simulink model "feedbackcontrol2"  (R2017b)
settings: Solver=VariableStepAuto  StartTime=0.0  StopTime=2000  MaxStep=0.04  RelTol=1e-3
values from neighbouring files (symbols this model uses):
  azi0 = 90/180*pi    (= 1.57079632679)    [MonteCarlo_f.m]    (also in MonteCarlo_l.m; MonteCarlo_s.m; calcu_delta.m = 0.174532925199; calcu_delta11.m)
  cd0 = 0.024    [flight_sim.m]
  cd1 = 7.24e-4    (= 0.000724)    [flight_sim.m]
  cd2 = 0.406    [flight_sim.m]
  cl0 = -0.2317    [flight_sim.m]
  cl1 = 0.0513    [flight_sim.m]
  cl2 = 0.2945    [flight_sim.m]
  delta_d = delta_d0(ii)    [MonteCarlo_f.m]    (also in MonteCarlo_l.m; MonteCarlo_s.m; calcu_delta11.m = -0.08; calcu_delta3.m = -0.079)
  delta_l = delta_l0(ii)    [MonteCarlo_f.m]    (also in MonteCarlo_l.m; MonteCarlo_s.m; calcu_delta3.m = 0.05)
  fpa0 = theta_0(ii)    [MonteCarlo_f.m]    (also in MonteCarlo_l.m; MonteCarlo_s.m; calcu_delta.m = -0.0349065850399; calcu_delta11.m = -0.0349065850399)
  hs = 7320    [constant.m]    (also in flight_sim.m)
  lat0 = 0    [MonteCarlo_f.m]    (also in MonteCarlo_l.m; MonteCarlo_s.m; calcu_delta.m; calcu_delta11.m)
  lon0 = 0    [MonteCarlo_f.m]    (also in MonteCarlo_l.m; MonteCarlo_s.m; calcu_delta.m; calcu_delta11.m)
  m = 92079.25    [constant.m]    (also in flight_sim.m = 907.2)
  r0 = r_0(ii)    [MonteCarlo_f.m]    (also in MonteCarlo_l.m; MonteCarlo_s.m; calcu_delta.m = Re+97500; calcu_delta11.m = Re+100000)
  Re = 6371393    [calcu_R.m]    (also in calcu_R2.m; calcu_c.m; constant.m = 6378145; flight_sim.m)
  rho0 = rho_0(ii)    [MonteCarlo_f.m]    (also in MonteCarlo_l.m; MonteCarlo_s.m; constant.m = 1.225; flight_sim.m = 1.225)
  S = 249.9    [constant.m]    (also in flight_sim.m = 0.484)
  solution = output.result.solution    [calcu_A_B.m]    (also in calcu_A_B1.m; calcu_A_B2.m; main_bank.m)
  V0 = V_0(ii)    [MonteCarlo_f.m]    (also in MonteCarlo_l.m; MonteCarlo_s.m; calcu_delta.m = 7900; calcu_delta11.m = 7900)
undefined symbols (not defined in the file or in its folder): Kdh, Kh, mu
settings Model: NumberOfSteps=500  Creator=ztyab  LastModifiedBy=ztyab
settings DataIOCC: SaveFormat=Array

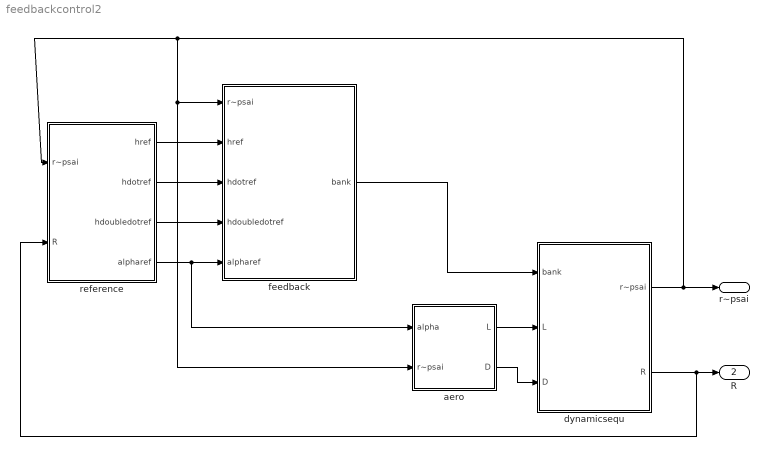
== system feedbackcontrol2 ==
  aero : Subsystem
  dynamicsequ : Subsystem
  feedback : Subsystem
  reference : Subsystem
  r~psai : Outport
  R : Outport  Port=2
  wires:
  aero/1(L) -> dynamicsequ/2(L)
  aero/2(D) -> dynamicsequ/3(D)
  reference/4(alpharef) -> aero/1(alpha), feedback/5(alpharef)
  reference/3(hdoubledotref) -> feedback/4(hdoubledotref)
  reference/1(href) -> feedback/2(href)
  reference/2(hdotref) -> feedback/3(hdotref)
  dynamicsequ/2(R) -> reference/2(R), R/1
  dynamicsequ/1(r~psai) -> feedback/1(r~psai), aero/2(r~psai), reference/1(r~psai), r~psai/1
  feedback/1(bank) -> dynamicsequ/1(bank)

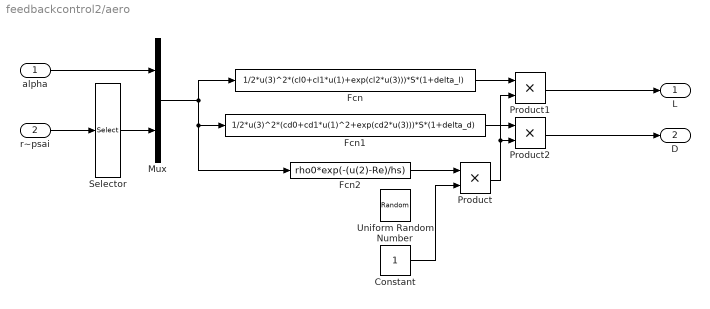
== system feedbackcontrol2/aero ==
  alpha : Inport
  r~psai : Inport  Port=2
  Constant : Constant
  Fcn : Fcn  Expr=1/2*u(3)^2*(cl0+cl1*u(1)+exp(cl2*u(3)))*S*(1+delta_l)
  Fcn1 : Fcn  Expr=1/2*u(3)^2*(cd0+cd1*u(1)^2+exp(cd2*u(3)))*S*(1+delta_d)
  Fcn2 : Fcn  Expr=rho0*exp(-(u(2)-Re)/hs)
  Mux : Mux  Inputs=2
  Product : Product
  Product1 : Product
  Product2 : Product
  Selector : Selector  InputPortWidth=6  IndexOptions=Index vector (dialog)  Indices=[1 4]  OutputSizes=1
  Uniform Random Number : UniformRandomNumber  Minimum=0.5  Maximum=1.5  SampleTime=0.01
  L : Outport
  D : Outport  Port=2
  wires:
  Mux/1 -> Fcn1/1, Fcn2/1, Fcn/1
  alpha/1 -> Mux/1
  r~psai/1 -> Selector/1
  Selector/1 -> Mux/2
  Fcn2/1 -> Product/1
  Product/1 -> Product1/2, Product2/2
  Fcn/1 -> Product1/1
  Fcn1/1 -> Product2/1
  Product1/1 -> L/1
  Product2/1 -> D/1
  Constant/1 -> Product/2

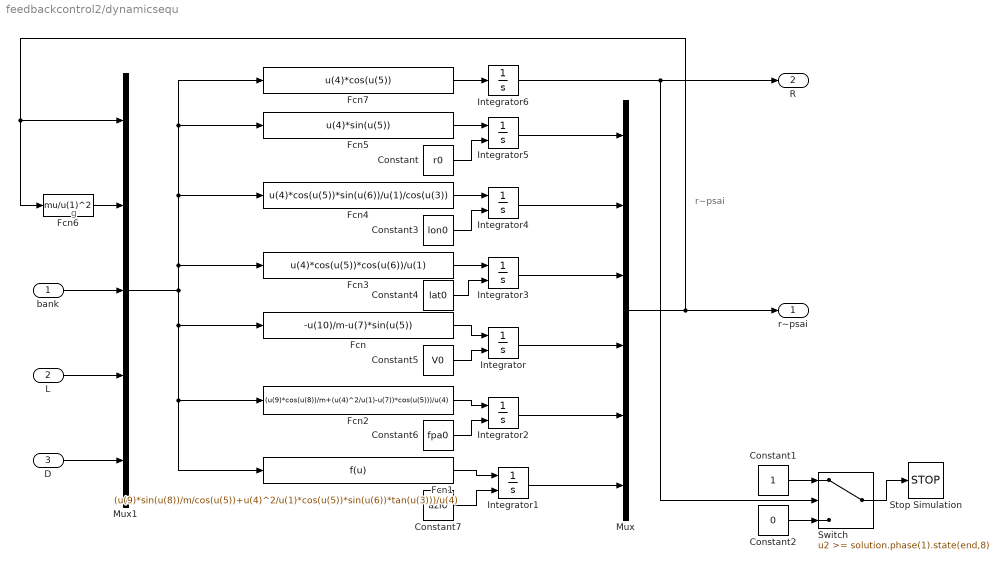
== system feedbackcontrol2/dynamicsequ ==
  note: g
  note: r~psai
  bank : Inport
  L : Inport  Port=2
  D : Inport  Port=3
  Constant : Constant  Value=r0
  Constant1 : Constant
  Constant2 : Constant  Value=0
  Constant3 : Constant  Value=lon0
  Constant4 : Constant  Value=lat0
  Constant5 : Constant  Value=V0
  Constant6 : Constant  Value=fpa0
  Constant7 : Constant  Value=azi0
  Fcn : Fcn  Expr=-u(10)/m-u(7)*sin(u(5))
  Fcn1 : Fcn  Expr=(u(9)*sin(u(8))/m/cos(u(5))+u(4)^2/u(1)*cos(u(5))*sin(u(6))*tan(u(3)))/u(4)
  Fcn2 : Fcn  Expr=(u(9)*cos(u(8))/m+(u(4)^2/u(1)-u(7))*cos(u(5)))/u(4)
  Fcn3 : Fcn  Expr=u(4)*cos(u(5))*cos(u(6))/u(1)
  Fcn4 : Fcn  Expr=u(4)*cos(u(5))*sin(u(6))/u(1)/cos(u(3))
  Fcn5 : Fcn  Expr=u(4)*sin(u(5))
  Fcn6 : Fcn  Expr=mu/u(1)^2
  Fcn7 : Fcn  Expr=u(4)*cos(u(5))
  Integrator : Integrator  InitialConditionSource=external  InitialCondition=7500
  Integrator1 : Integrator  InitialConditionSource=external  InitialCondition=10*pi/180
  Integrator2 : Integrator  InitialConditionSource=external  InitialCondition=-2/180*pi
  Integrator3 : Integrator  InitialConditionSource=external
  Integrator4 : Integrator  InitialConditionSource=external
  Integrator5 : Integrator  InitialConditionSource=external  InitialCondition=95000+6371393
  Integrator6 : Integrator
  Mux : Mux  Inputs=6
  Mux1 : Mux  Inputs=5
  Stop Simulation : Stop
  Switch : Switch  Threshold=solution.phase(1).state(end,8)
  r~psai : Outport
  R : Outport  Port=2
  wires:
  Fcn6/1 -> Mux1/2
  Mux/1 -> Fcn6/1, Mux1/1, r~psai/1
  Fcn1/1 -> Integrator1/1
  Integrator1/1 -> Mux/6
  Fcn2/1 -> Integrator2/1
  Integrator4/1 -> Mux/2
  Fcn/1 -> Integrator/1
  Integrator2/1 -> Mux/5
  Fcn4/1 -> Integrator4/1
  Integrator3/1 -> Mux/3
  Fcn3/1 -> Integrator3/1
  Integrator/1 -> Mux/4
  Fcn5/1 -> Integrator5/1
  Integrator5/1 -> Mux/1
  L/1 -> Mux1/4
  D/1 -> Mux1/5
  bank/1 -> Mux1/3
  Mux1/1 -> Fcn1/1, Fcn2/1, Fcn/1, Fcn4/1, Fcn7/1, Fcn5/1, Fcn3/1
  Fcn7/1 -> Integrator6/1
  Integrator6/1 -> Switch/2, R/1
  Constant2/1 -> Switch/3
  Constant1/1 -> Switch/1
  Switch/1 -> Stop Simulation/1
  Constant/1 -> Integrator5/2
  Constant3/1 -> Integrator4/2
  Constant4/1 -> Integrator3/2
  Constant5/1 -> Integrator/2
  Constant6/1 -> Integrator2/2
  Constant7/1 -> Integrator1/2

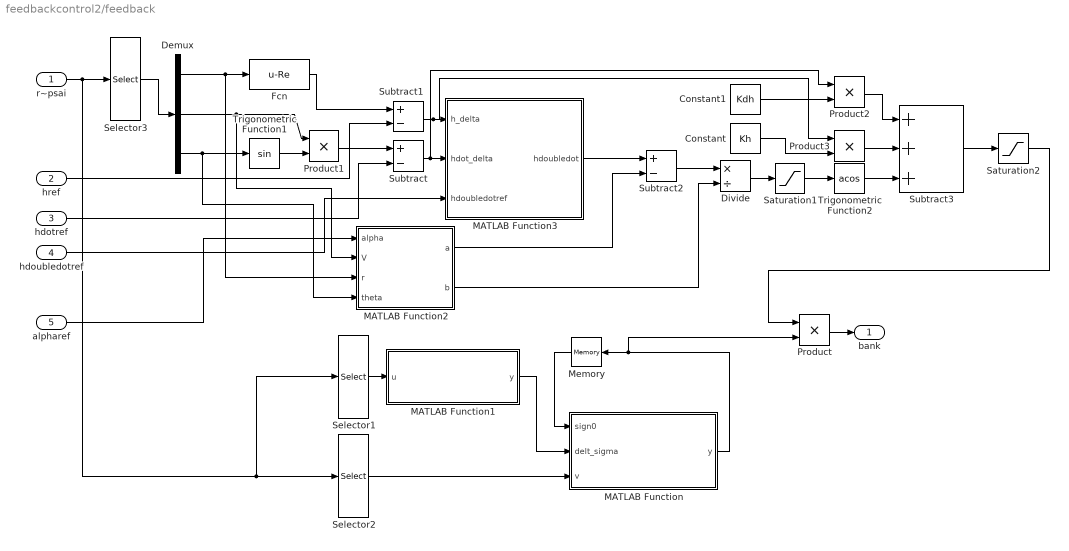
== system feedbackcontrol2/feedback ==
  r~psai : Inport
  href : Inport  Port=2
  hdotref : Inport  Port=3
  hdoubledotref : Inport  Port=4
  alpharef : Inport  Port=5
  Constant : Constant  Value=Kh
  Constant1 : Constant  Value=Kdh
  Demux : Demux  Outputs=3
  Divide : Product  Inputs=*/
  Fcn : Fcn  Expr=u-Re
  MATLAB Function : MATLAB Function  TreatAsAtomicUnit=on
  MATLAB Function1 : MATLAB Function  TreatAsAtomicUnit=on
  MATLAB Function2 : MATLAB Function  TreatAsAtomicUnit=on
  MATLAB Function3 : MATLAB Function  TreatAsAtomicUnit=on
  Memory : Memory
  Product{,1..3} (4 alike) : Product
  Saturation1 : Saturate  UpperLimit=1  LowerLimit=cos(89/180*pi)
  Saturation2 : Saturate  UpperLimit=89/180*pi  LowerLimit=0
  Selector1 : Selector  InputPortWidth=6  IndexOptions=Index vector (dialog)  Indices=[2 3 6]  OutputSizes=1
  Selector2 : Selector  InputPortWidth=6  IndexOptions=Index vector (dialog)  Indices=[4]  OutputSizes=1
  Selector3 : Selector  InputPortWidth=6  IndexOptions=Index vector (dialog)  Indices=[1 4 5]  OutputSizes=1
  Subtract : Sum  Inputs=+-
  Subtract1 : Sum  Inputs=+-
  Subtract2 : Sum  Inputs=+-
  Subtract3 : Sum  Inputs=+++
  Trigonometric Function1 : Trigonometry
  Trigonometric Function2 : Trigonometry  Operator=acos
  bank : Outport
  wires:
  Memory/1 -> MATLAB Function/1(sign0)
  Selector2/1 -> MATLAB Function/3(v)
  MATLAB Function1/1(y) -> MATLAB Function/2(delt_sigma)
  r~psai/1 -> Selector2/1, Selector1/1, Selector3/1
  MATLAB Function/1(y) -> Product/2, Memory/1
  Product/1 -> bank/1
  Selector1/1 -> MATLAB Function1/1(u)
  Selector3/1 -> Demux/1
  Demux/1 -> MATLAB Function2/3(r), Fcn/1
  Trigonometric Function1/1 -> Product1/2
  Product1/1 -> Subtract/1
  hdotref/1 -> Subtract/2
  Fcn/1 -> Subtract1/1
  href/1 -> Subtract1/2
  Subtract1/1 -> Product3/1, MATLAB Function3/1(h_delta)
  Subtract/1 -> Product2/1, MATLAB Function3/2(hdot_delta)
  hdoubledotref/1 -> MATLAB Function3/3(hdoubledotref)
  alpharef/1 -> MATLAB Function2/1(alpha)
  Demux/2 -> MATLAB Function2/2(V), Product1/1
  Demux/3 -> MATLAB Function2/4(theta), Trigonometric Function1/1
  MATLAB Function3/1(hdoubledot) -> Subtract2/1
  MATLAB Function2/1(a) -> Subtract2/2
  Subtract2/1 -> Divide/1
  MATLAB Function2/2(b) -> Divide/2
  Divide/1 -> Saturation1/1
  Saturation1/1 -> Trigonometric Function2/1
  Trigonometric Function2/1 -> Subtract3/3
  Product3/1 -> Subtract3/2
  Product2/1 -> Subtract3/1
  Constant/1 -> Product3/2
  Constant1/1 -> Product2/2
  Subtract3/1 -> Saturation2/1
  Saturation2/1 -> Product/1

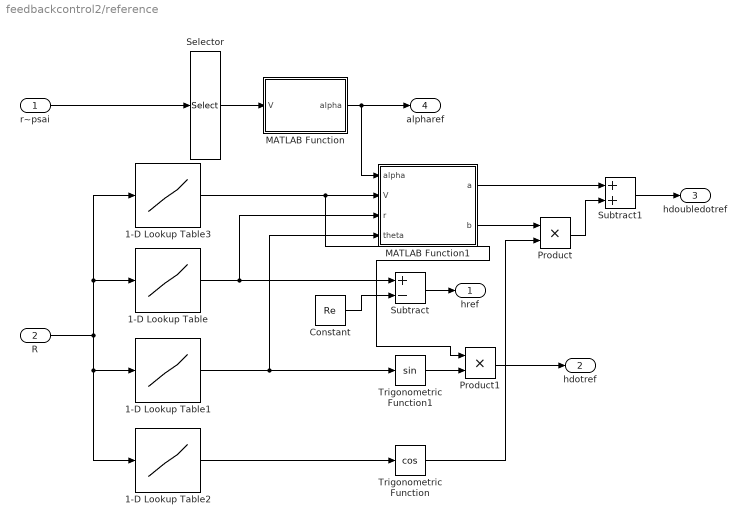
== system feedbackcontrol2/reference ==
  r~psai : Inport
  R : Inport  Port=2
  1-D Lookup Table : Lookup_n-D  NumberOfTableDimensions=1  BreakpointsForDimension1=solution.phase(1).state(:,8)  Table=solution.phase(1).state(:,1)  InterpMethod=Cubic spline  ExtrapMethod=Cubic spline  InternalRulePriority=Speed  RndMeth=Simplest  InputSameDT=on
  1-D Lookup Table1 : Lookup_n-D  NumberOfTableDimensions=1  BreakpointsForDimension1=solution.phase(1).state(:,8)  Table=solution.phase(1).state(:,5)  InterpMethod=Cubic spline  ExtrapMethod=Cubic spline  InternalRulePriority=Speed  RndMeth=Simplest  InputSameDT=on
  1-D Lookup Table2 : Lookup_n-D  NumberOfTableDimensions=1  BreakpointsForDimension1=solution.phase(1).state(:,8)  Table=solution.phase(1).state(:,7)  InterpMethod=Cubic spline  ExtrapMethod=Cubic spline  InternalRulePriority=Speed  RndMeth=Simplest  InputSameDT=on
  1-D Lookup Table3 : Lookup_n-D  NumberOfTableDimensions=1  BreakpointsForDimension1=solution.phase(1).state(:,8)  Table=solution.phase(1).state(:,4)  InterpMethod=Cubic spline  ExtrapMethod=Cubic spline  InternalRulePriority=Speed  RndMeth=Simplest  InputSameDT=on
  Constant : Constant  Value=Re
  MATLAB Function : MATLAB Function  TreatAsAtomicUnit=on
  MATLAB Function1 : MATLAB Function  TreatAsAtomicUnit=on
  Product : Product
  Product1 : Product
  Selector : Selector  InputPortWidth=6  IndexOptions=Index vector (dialog)  Indices=[4]  OutputSizes=1
  Subtract : Sum  Inputs=+-
  Subtract1 : Sum
  Trigonometric Function : Trigonometry  Operator=cos
  Trigonometric Function1 : Trigonometry
  href : Outport
  hdotref : Outport  Port=2
  hdoubledotref : Outport  Port=3
  alpharef : Outport  Port=4
  wires:
  r~psai/1 -> Selector/1
  MATLAB Function/1(alpha) -> alpharef/1, MATLAB Function1/1(alpha)
  Selector/1 -> MATLAB Function/1(V)
  Subtract/1 -> href/1
  Constant/1 -> Subtract/2
  MATLAB Function1/1(a) -> Subtract1/1
  MATLAB Function1/2(b) -> Product/1
  Product/1 -> Subtract1/2
  Trigonometric Function/1 -> Product/2
  Subtract1/1 -> hdoubledotref/1
  Trigonometric Function1/1 -> Product1/2
  Product1/1 -> hdotref/1
  1-D Lookup Table/1 -> MATLAB Function1/3(r), Subtract/1
  1-D Lookup Table1/1 -> MATLAB Function1/4(theta), Trigonometric Function1/1
  1-D Lookup Table2/1 -> Trigonometric Function/1
  R/1 -> 1-D Lookup Table2/1, 1-D Lookup Table1/1, 1-D Lookup Table3/1, 1-D Lookup Table/1
  1-D Lookup Table3/1 -> MATLAB Function1/2(V), Product1/1

== matlab function feedbackcontrol2/feedback/MATLAB Function1 ==
  data: u input; y output
function y = fcn(u)
lambda=u(1);
phi=u(2);
sigma=u(3);
lambdaf=48*pi/180;
phif=60*pi/180;
if phi>phif
    sigma_t=pi-asin(cos(phif)*sin(lambdaf-lambda)/sin(acos(sin(phif)*sin(phi)+cos(phif)*cos(phi)*cos(lambdaf-lambda))));
else
    sigma_t=asin(cos(phif)*sin(lambdaf-lambda)/sin(acos(sin(phif)*sin(phi)+cos(phif)*cos(phi)*cos(lambdaf-lambda))));
end
y=sigma-sigma_t;
end

== matlab function feedbackcontrol2/reference/MATLAB Function ==
  data: V input; alpha output
function alpha = calcu_alpha(V)

v1=6500;
v2=5000;
alpha0=20*pi/180;
alphaf=10*pi/180;
alpha=(alpha0.*(V>v1)+((V-v1)*(alphaf-alpha0)/(v2-v1)+alpha0).*(V<=v1&V>=v2)+alphaf.*(V<v2));

end

== matlab function feedbackcontrol2/feedback/MATLAB Function ==
  data: sign0 input; y output; delt_sigma input; v input
function y = fcn(sign0,delt_sigma,v)

%#codegen
delt_sigma1=15/180*pi;
delt_sigma2=30/180*pi;
delt_sigma3=5/180*pi;
if (v>=6000)
    if (delt_sigma>delt_sigma1)
        sign=-1;
    elseif (delt_sigma<=delt_sigma1)&&(delt_sigma>=-delt_sigma1)
        sign=sign0;
    else 
        sign=1;
    end
elseif (4000<=v&v<6000)
    if (delt_sigma>delt_sigma2)
        sign=-1;
    elseif (delt_sigma<=delt_sigma2)&&(delt_sigma>=-delt_sigma2)
        sign=sign0;
    else 
        sign=1;
    end
elseif (3000<=v&&v<4000)
    delt=delt_sigma3+(delt_sigma2-delt_sigma3)/(4000-3000)*(v-3000);
    if (delt_sigma>delt)
        sign=-1;
    elseif (delt_sigma<=delt)&&(delt_sigma>=-delt)
        sign=sign0;
    else 
        sign=1;
    end  
else
    if (delt_sigma>delt_sigma3)
        sign=-1;
    elseif (delt_sigma<=delt_sigma3)&&(delt_sigma>=-delt_sigma3)
        sign=sign0;
    else 
        sign=1;
    end  
end
if(sign0==0)
    sign=1;
end
y =sign;
end

== matlab function feedbackcontrol2/reference/MATLAB Function1 ==
  data: alpha input; a output; V input; r input; theta input; b output
function [a,b] = fcn(alpha,V,r,theta)
m=498.95;
S=0.113;
cd2 = -0.05119/340;
cd1 = 0.001944*57.3^2;
cd0 = -0.03795;
cl2 = 0.0017/340;
cl1 = 0.07412*57.3;
cl0 = -0.998;
rho0=1.225;
g0=9.81;
Re=6371393;
mu=g0*Re^2;
hs=7320;
Cl=exp(cl2*V)+cl1*alpha+cl0;
Cd=exp(cd2*V)+cd1*alpha.^2+cd0;
rho=rho0.*exp(-(r-Re)./hs);
q=1/2*rho.*V.^2;
L=q.*Cl.*S;
D=q.*Cd.*S;
g=mu./r.^2;

a=-D/m*sin(theta)-g+V^2*cos(theta)^2/r;
b=L*cos(theta)/m;


end

== matlab function feedbackcontrol2/feedback/MATLAB Function2 ==
  data: alpha input; a output; V input; r input; theta input; b output
function [a,b] = fcn(alpha,V,r,theta)
m=498.95;
S=0.113;
cd2 = -0.05119/340;
cd1 = 0.001944*57.3^2;
cd0 = -0.03795;
cl2 = 0.0017/340;
cl1 = 0.07412*57.3;
cl0 = -0.998;
rho0=1.225;
g0=9.81;
Re=6371393;
mu=g0*Re^2;
hs=7320;
Cl=(exp(cl2*V)+cl1*alpha+cl0);
Cd=(exp(cd2*V)+cd1*alpha.^2+cd0);
rho=rho0.*exp(-(r-Re)./hs);
q=1/2*rho.*V.^2;
L=q.*Cl.*S;
D=q.*Cd.*S;
g=mu./r.^2;

a=-D/m*sin(theta)-g+V^2*cos(theta)^2/r;
b=L*cos(theta)/m;


end

== matlab function feedbackcontrol2/feedback/MATLAB Function3 ==
  data: h_delta input; hdoubledot output; hdot_delta input; hdoubledotref input
function hdoubledot = fcn(h_delta,hdot_delta,hdoubledotref)
k=0.707;
w=0.03;
hdoubledot=hdoubledotref-2*k*w*hdot_delta-w^2*h_delta;
end
